simulink model "FYP"  (R2017a)
settings: Solver=VariableStepAuto  StartTime=0.0  StopTime=499  RelTol=1e-3  EnableMultiTasking=on
values from neighbouring files (symbols this model uses):
  acc = zeros(3,N)    [FYP_physical.m]    (also in FYP_virtual.m = zeros(6,size(x,2)); newsys3.m = zeros(6,size(x,2)))
  K = P*sysd.C'/(sysd.C*P*sysd.C'+R)    [FYP_physical.m]    (also in FYP_virtual.m)
  Plantd = c2d(Plant,0.05)    [FYP_virtual.m]
  sysd = c2d(sys,0.01/3)    [FYP_physical.m]    (also in FYP_virtual.m = c2d(sys,0.05))
  v1 = zeros(12,N)    [FYP_physical.m]    (also in FYP_virtual.m)
  v2 = yv - y    [FYP_physical.m]    (also in FYP_virtual.m = (yv - y))
  x0 = [w(:,1); (w(1:3,2)-w(1:3,1))/h; v(:,1)]    [FYP_physical.m]    (also in FYP_virtual.m = [w(:,1) ; v(:,1)]; newsys3.m = [w(:,1) ; v(:,1)])
  y0 = [w(:,1); v(:,1); u(:,1)]    [FYP_physical.m]    (also in FYP_virtual.m = [w(:,1) ; v(4,1); v(5,1); v(6,1); u(1,1); u(2,1); u(3,1)])
settings Model: Creator=ebm13  LastModifiedBy=eirillbm
settings OptimizationCC: LifeSpan=inf
settings DebuggingCC: SFUnexpectedBacktrackingDiag=warning  SFNoUnconditionalDefaultTransitionDiag=warning  SFExecutionAtInitializationDiag=none
settings GRTTargetCC: TargetLangStandard=C89/C90 (ANSI)  GeneratePreprocessorConditionals=Disable all
settings ConfigComp: CovMetricSettings=dw  CovHtmlReporting=on  CovSaveCumulativeToWorkspaceVar=on  CovSaveSingleToWorkspaceVar=on  CovExternalEMLEnable=off

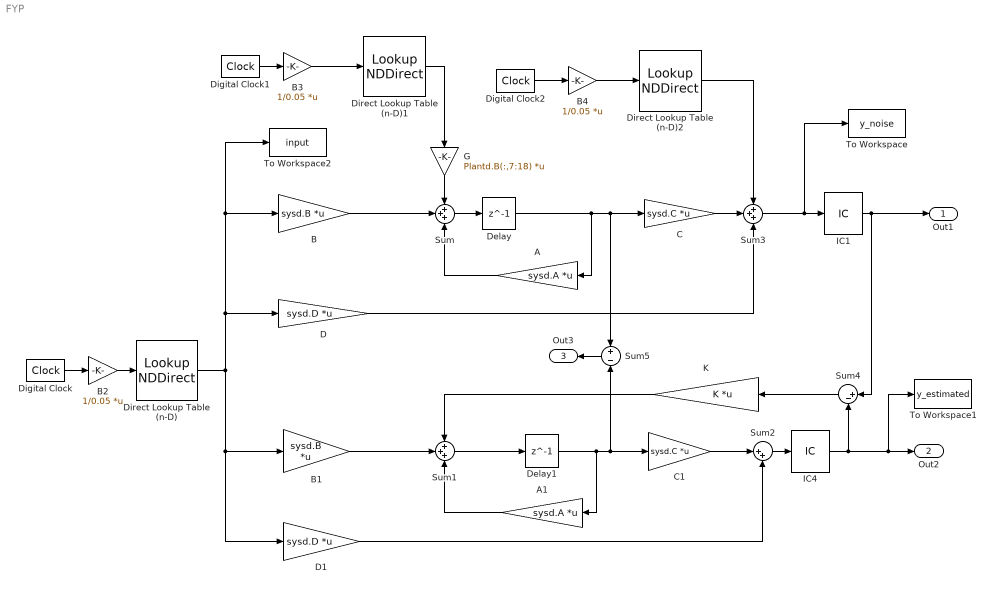
== system FYP ==
  A : Gain  Gain=sysd.A  Multiplication=Matrix(K*u)
  A1 : Gain  Gain=sysd.A  Multiplication=Matrix(K*u)
  B : Gain  Gain=sysd.B  Multiplication=Matrix(K*u)
  B1 : Gain  Gain=sysd.B  Multiplication=Matrix(K*u)
  B2 : Gain  Gain=1/0.05  Multiplication=Matrix(K*u)
  B3 : Gain  Gain=1/0.05  Multiplication=Matrix(K*u)
  B4 : Gain  Gain=1/0.05  Multiplication=Matrix(K*u)
  C : Gain  Gain=sysd.C  Multiplication=Matrix(K*u)
  C1 : Gain  Gain=sysd.C  Multiplication=Matrix(K*u)
  D : Gain  Gain=sysd.D  Multiplication=Matrix(K*u)
  D1 : Gain  Gain=sysd.D  Multiplication=Matrix(K*u)
  Delay : Delay  DelayLength=1  InitialCondition=x0
  Delay1 : Delay  DelayLength=1  InitialCondition=x0
  Digital Clock : DigitalClock  SampleTime=0.05
  Digital Clock1 : DigitalClock  SampleTime=0.05
  Digital Clock2 : DigitalClock  SampleTime=0.05
  Direct Lookup Table (n-D) : LookupNDDirect  InputsSelectThisObjectFromTable=Column  Table=acc
  Direct Lookup Table (n-D)1 : LookupNDDirect  InputsSelectThisObjectFromTable=Column  Table=v1
  Direct Lookup Table (n-D)2 : LookupNDDirect  InputsSelectThisObjectFromTable=Column  Table=v2
  G : Gain  Gain=Plantd.B(:,7:18)  Multiplication=Matrix(K*u)
  IC1 : InitialCondition  Value=y0
  IC4 : InitialCondition  Value=y0
  K : Gain  Gain=K  Multiplication=Matrix(K*u)
  Sum : Sum  Inputs=+++
  Sum1 : Sum  Inputs=+++
  Sum2 : Sum  Inputs=|++
  Sum3 : Sum  Inputs=+++
  Sum4 : Sum  Inputs=|+-
  Sum5 : Sum  Inputs=+|-
  To Workspace : ToWorkspace  VariableName=y_noise  SaveFormat=Timeseries  SampleTime=-1
  To Workspace1 : ToWorkspace  VariableName=y_estimated  SaveFormat=Timeseries  SampleTime=-1
  To Workspace2 : ToWorkspace  VariableName=input  SaveFormat=Timeseries  SampleTime=-1
  Out1 : Outport
  Out2 : Outport  Port=2
  Out3 : Outport  Port=3
  wires:
  B/1 -> Sum/2
  Sum/1 -> Delay/1
  A/1 -> Sum/3
  B1/1 -> Sum1/2
  Sum1/1 -> Delay1/1
  A1/1 -> Sum1/3
  C/1 -> Sum3/2
  D/1 -> Sum3/3
  Sum3/1 -> To Workspace/1, IC1/1
  Sum4/1 -> K/1
  K/1 -> Sum1/1
  Direct Lookup Table (n-D)2/1 -> Sum3/1
  B3/1 -> Direct Lookup Table (n-D)1/1
  C1/1 -> Sum2/1
  D1/1 -> Sum2/2
  Digital Clock/1 -> B2/1
  Direct Lookup Table (n-D)/1 -> To Workspace2/1, B/1, D/1, D1/1, B1/1
  B2/1 -> Direct Lookup Table (n-D)/1
  Direct Lookup Table (n-D)1/1 -> G/1
  Digital Clock1/1 -> B3/1
  Digital Clock2/1 -> B4/1
  B4/1 -> Direct Lookup Table (n-D)2/1
  Sum2/1 -> IC4/1
  Delay/1 -> C/1, Sum5/1, A/1
  IC1/1 -> Sum4/1, Out1/1
  Delay1/1 -> Sum5/2, C1/1, A1/1
  IC4/1 -> Sum4/2, To Workspace1/1, Out2/1
  Sum5/1 -> Out3/1
  G/1 -> Sum/1
